simulink library "PC_Simulator_Lib"  (Simulink 8.2)
settings: Solver=ode45  StartTime=0.0  StopTime=10.0  RelTol=1e-3
values from neighbouring files (symbols this model uses):
  data = [r1 r2 r3 r4 L1 L2 L3 L4]    [strasse_Bedatung_HNI_ITI.m]
  distSameLane = 60    [InitialisationsEnv.m]
  eng_speed = [0 60 120 180 240 300 360 420 480 540 600 660 ... (101 elements, 1x101)]    [engine_table.mat]    (also in motor_parameter_calc.m = omega)
  Heading_init = 0    [Start.m]
  inertiaLateral = 25*(radiusWheel)^2    (= 4.129024)    [Start.m]
  laneWidth = 3.6    [InitialisationsEnv.m]    (also in strasse_Bedatung_HNI_ITI.m)
  omega_engine = [0.000000 150.000000 500.000000 1000.000000 1500.000000 2000.000000 2500.000000 3000.000000 3500.000000 4000.000000 4500.000000 5000.000000 5500.000000 6000.000000]    [friction_tables.m]
  omega_max = 6000    [engine_table.mat]    (also in motor_parameter_calc.m)
  omega_wheel = [0 20 40 60 80 100 122 143.7 164]    [friction_tables.m]
  para_Fellow_8_Points = ADAS.Fellow_8_Points    [ADAS_parameters.m]
  position_start_x = [x1 x2 x3 x4 x5 x6 x7]    [strasse_Bedatung_HNI_ITI.m]
  position_start_y = [y1 y2 y3 y4 y5 y6 y7]    [strasse_Bedatung_HNI_ITI.m]
  rad3rdLine = 57.2    [InitialisationsEnv.m]    (also in strasse_Bedatung_HNI_ITI.m)
  radiusWheel = 16*2.54/100    (= 0.4064)    [Start.m]
  s_values = [S1 S2 S3 S4 S5 S6 S7]    [strasse_Bedatung_HNI_ITI.m]
  segmentLimits = [segment1EndThirdLine                   segment2EndThirdLine                   segment3EndThirdLine                   segment4EndThirdLine                   segment5EndThirdLine                   segment6EndThirdLine                   segment7EndThirdLine                   segment8EndThirdLine                   ]    [InitialisationsEnv.m]    (also in strasse_Bedatung_HNI_ITI.m)
  setPosT = [-1.8 -5.4 -1.8 -5.4 -1.8 -5.4 -1.8 -5.4 -1.8 -5.4]    [InitialisationsEnv.m]
  torque = [297.089227105 300.997600937 304.800343044 308.497453426 312.088932082 315.574779014 318.95499422 322.229577701 325.398529457 328.461849487 331.419537793 334.271594373 ... (101 elements, 1x101)]    [engine_table.mat]    (also in motor_parameter_calc.m = g)
  Torque_lost = [0.000000 -8.777780 -15.000000 -26.800000 -29.600000 -32.700000 -35.900000 -39.300000 -42.800000 -46.500000 -50.300000 -54.300000 -58.500000 -62.800000 ]*0.6    [friction_tables.m]
  Torque_lost_wheel = [0.8 0.8 0.75 0.7 0.4 0.3 0.2 0.07 0.07]*0.2    [friction_tables.m]
  X_init = 0    [Start.m]
  Y_init = 1.8    [Start.m]
  Z_init = 0    [Start.m]
undefined symbols (not defined in the file or in its folder): Acc_Pedal, ADAS, Brake_Pedal, Joystick, Newton, Para, Raphson, Standard_Devices, Steering_Wheel_Angle, UDP_Protocol
libraries: simulink x43, rtwinlib x7, dspnetwork x2, simulink_extras x1, vrlib x1
(part 5 of 13)

== system PC_Simulator_Lib/ADAS/Decision_Making_ADAS/Maping_Input ==
  Feedback_ADAS : Inport
  Feedback_Simulationsumgebung : Inport  Port=2
  Abs : Abs
  Bus Selector : BusSelector  OutputSignals=Vehicle_Dynamics.position_CoG.x_CoG[m],Vehicle_Dynamics.position_CoG.y_CoG[m],Vehicle_Dynamics.Oriantation_CoG.Yaw_Angle,Vehicle_Dynamics.Vx_COG[m|s],Environment.Main_Vehicle.t_VUT[m]
  Bus Selector1 : BusSelector  OutputSignals=Unser_Interface_ADAS.ACC.ACC_State,Unser_Interface_ADAS.Pilotiertes_Fahren.Pilotiertes_Fahren_State,Unser_Interface_ADAS.Emergency_Brake.Emergency_Brake_State,Unser_Interface_ADAS.Emergency_Steering.Emergency_Steering_State,Unser_Interface_ADAS.ACC.ACC_Set_Speed[m|s],Unser_Interface_ADAS.ACC.ACC_Time_Gap[s],Sensors_ADAS.Sensors_Front_Out.Object_Detected_In_Lane[bool],Sensors_ADAS.Sensors_Front_Out.Distance[m],Sensors_ADAS.Sensors_Front_Out.Relative_Velocity[m|s],Sensors_ADAS.Sensors_Front_Out.direction_delta_T_available,Sensors_ADAS.Sensors_Front_Out.Lateral_distance_available[m],Sensors_ADAS.Sensors_Front_Out.Heading_Angle_Difference[deg]
  Memory : Memory
  signals_manipulation : Subsystem
  x_CoG_VUT[m] : Outport
  y_CoG_VUT[m] : Outport  Port=2
  yaw_VUT[rad] : Outport  Port=3
  Vx_CoG_VUT[m|s] : Outport  Port=4
  Active_System : Outport  Port=5
  V_User_Set_Speed[m|s] : Outport  Port=6
  Time_Gap[s] : Outport  Port=7
  Object_Inlane[bool] : Outport  Port=8
  Distance_2_Object_Sensor[m] : Outport  Port=9
  v_relative_Sensor[m|s] : Outport  Port=10
  T_current[m] : Outport  Port=11
  Direction_delta_T_Available : Outport  Port=12
  Lateral_Distance_Available[m] : Outport  Port=13
  Heading_Angle_Difference_Absolute[deg] : Outport  Port=14
  wires:
  Abs/1 -> Heading_Angle_Difference_Absolute[deg]/1
  Bus Selector1/12 -> Abs/1  "<Heading_Angle_Difference[deg]>"
  Feedback_Simulationsumgebung/1 -> Bus Selector/1
  Bus Selector/3 -> yaw_VUT[rad]/1  "<Yaw_Angle>"
  Bus Selector/4 -> Vx_CoG_VUT[m|s]/1  "<Vx_COG[m|s]>"
  Bus Selector/2 -> y_CoG_VUT[m]/1  "<y_CoG[m]>"
  Bus Selector/1 -> x_CoG_VUT[m]/1  "<x_CoG[m]>"
  Feedback_ADAS/1 -> Bus Selector1/1
  Bus Selector1/6 -> Time_Gap[s]/1  "<ACC_Time_Gap[s]>"
  Bus Selector1/5 -> Memory/1  "<ACC_Set_Speed[m|s]>"
  Memory/1 -> V_User_Set_Speed[m|s]/1
  Bus Selector1/1 -> signals_manipulation/1(ACC_State)  "<ACC_State>"
  Bus Selector1/7 -> Object_Inlane[bool]/1  "<Object_Detected_In_Lane[bool]>"
  Bus Selector1/8 -> Distance_2_Object_Sensor[m]/1  "<Distance[m]>"
  Bus Selector1/9 -> v_relative_Sensor[m|s]/1  "<Relative_Velocity[m|s]>"
  Bus Selector/5 -> T_current[m]/1  "<t_VUT[m]>"
  Bus Selector1/2 -> signals_manipulation/2(Pilotiertes_Fahren_State)  "<Pilotiertes_Fahren_State>"
  signals_manipulation/1(Active_System) -> Active_System/1
  Bus Selector1/3 -> signals_manipulation/3(Emergency_Brkae_State)  "<Emergency_Brake_State>"
  Bus Selector1/10 -> Direction_delta_T_Available/1  "<direction_delta_T_available>"
  Bus Selector1/11 -> Lateral_Distance_Available[m]/1  "<Lateral_distance_available[m]>"
  Bus Selector1/4 -> signals_manipulation/4(Emergency_Steering_State)  "<Emergency_Steering_State>"

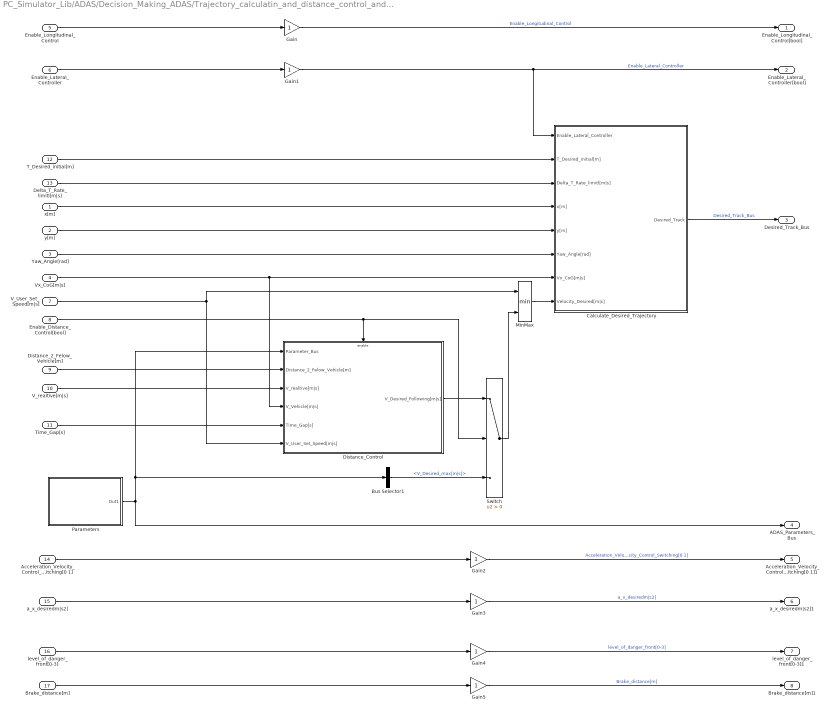
== system PC_Simulator_Lib/ADAS/Decision_Making_ADAS/Trajectory_calculatin_and_distance_control_and output_maping ==
  x[m] : Inport
  y[m] : Inport  Port=2
  Yaw_Angle[rad] : Inport  Port=3
  Vx_CoG[m|s] : Inport  Port=4
  Enable_Longitudinal_Control : Inport  Port=5
  Enable_Lateral_Controller : Inport  Port=6
  V_User_Set_Speed[m|s] : Inport  Port=7
  Enable_Distance_Control[bool] : Inport  Port=8
  Distance_2_Felow_Vehicle[m] : Inport  Port=9
  V_realtive[m|s] : Inport  Port=10
  Time_Gap[s] : Inport  Port=11
  T_Desired_initial[m] : Inport  Port=12
  Delta_T_Rate_limitl[m|s] : Inport  Port=13
  Acceleration_Velocity_Control_Switching[0 1] : Inport  Port=14
  a_x_desiredm|s2] : Inport  Port=15
  level_of_danger_front[0-3] : Inport  Port=16
  Brake_distance[m] : Inport  Port=17
  Bus Selector1 : BusSelector  OutputSignals=V_Desired_max[m|s]
  Calculate_Desired_Trajectory : Subsystem
  Distance_Control : Subsystem
  Gain{,1..5} (6 alike) : Gain
  MinMax : MinMax  Inputs=2
  Parameters : Subsystem
  Switch : Switch  Criteria=u2 > Threshold
  Enable_Longitudinal_Control[bool] : Outport
  Enable_Lateral_Controller[bool] : Outport  Port=2
  Desired_Track_Bus : Outport  Port=3
  ADAS_Parameters_Bus : Outport  Port=4
  Acceleration_Velocity_Control_Switching[0 1]1 : Outport  Port=5
  "a_x_desiredm|s2]1 " : Outport  Port=6
  level_of_danger_front[0-3]1 : Outport  Port=7
  Brake_distance[m]1 : Outport  Port=8
  wires:
  Brake_distance[m]/1 -> Gain5/1
  Gain5/1 -> Brake_distance[m]1/1  "Brake_distance[m]"
  Gain4/1 -> level_of_danger_front[0-3]1/1  "level_of_danger_front[0-3]"
  level_of_danger_front[0-3]/1 -> Gain4/1
  Enable_Lateral_Controller/1 -> Gain1/1
  V_realtive[m|s]/1 -> Distance_Control/3(V_realtive[m|s])
  V_User_Set_Speed[m|s]/1 -> MinMax/1, Distance_Control/6(V_User_Set_Speed[m|s])
  T_Desired_initial[m]/1 -> Calculate_Desired_Trajectory/2(T_Desired_initial[m])
  Delta_T_Rate_limitl[m|s]/1 -> Calculate_Desired_Trajectory/3(Delta_T_Rate_limitl[m|s])
  Enable_Longitudinal_Control/1 -> Gain/1
  Calculate_Desired_Trajectory/1(Desired_Track) -> Desired_Track_Bus/1  "Desired_Track_Bus"
  MinMax/1 -> Calculate_Desired_Trajectory/8(Velocity_Desired[m|s])
  Distance_Control/1(V_Desired_Following[m|s]) -> Switch/1
  Enable_Distance_Control[bool]/1 -> Switch/2, Distance_Control/Enable
  Bus Selector1/1 -> Switch/3  "<V_Desired_max[m|s]>"
  Switch/1 -> MinMax/2
  Time_Gap[s]/1 -> Distance_Control/5(Time_Gap[s])
  x[m]/1 -> Calculate_Desired_Trajectory/4(x[m])
  y[m]/1 -> Calculate_Desired_Trajectory/5(y[m])
  Vx_CoG[m|s]/1 -> Calculate_Desired_Trajectory/7(Vx_CoG[m|s]), Distance_Control/4(V_Vehicle[m|s])
  Yaw_Angle[rad]/1 -> Calculate_Desired_Trajectory/6(Yaw_Angle[rad])
  Parameters/1(Out1) -> ADAS_Parameters_Bus/1, Distance_Control/1(Parameter_Bus), Bus Selector1/1
  Distance_2_Felow_Vehicle[m]/1 -> Distance_Control/2(Distance_2_Felow_Vehicle[m])
  Gain/1 -> Enable_Longitudinal_Control[bool]/1  "Enable_Longitudinal_Control"
  Gain1/1 -> Enable_Lateral_Controller[bool]/1, Calculate_Desired_Trajectory/1(Enable_Lateral_Controller)  "Enable_Lateral_Controller"
  Acceleration_Velocity_Control_Switching[0 1]/1 -> Gain2/1
  Gain2/1 -> Acceleration_Velocity_Control_Switching[0 1]1/1  "Acceleration_Velocity_Control_Switching[0 1]"
  a_x_desiredm|s2]/1 -> Gain3/1
  Gain3/1 -> "a_x_desiredm|s2]1 "/1  "a_x_desiredm|s2]"

== system PC_Simulator_Lib/ADAS/Execution_ADAS/Input_Interface ==
  Feedback_ADAS : Inport
  Feedback_Simulationsumgebung : Inport  Port=2
  Bus Selector : BusSelector  OutputSignals=Vehicle_Dynamics.ax_COG[m|s2],Vehicle_Dynamics.Vx_COG[m|s],Drive_Train.Omega_4_Wheels[rad|s],Drive_Train.Omega_Engine[rad|s],Drive_Train.Gearbox_Gear_Ratio,Driver_Interface.Acc_Pedal_norm,Driver_Interface.Brake_Pedal_norm,Driver_Interface.Steering_wheel_norm,Vehicle_Dynamics.Vy_COG[m|s],Vehicle_Dynamics.Oriantation_CoG.Yaw_Angle,Vehicle_Dynamics.Yaw_Rate[rad|s],Vehicle_Dynamics.position_CoG.x_CoG[m],Vehicle_Dynamics.position_CoG.y_CoG[m]
  Bus Selector1 : BusSelector  OutputSignals=Decision_Making_ADAS.Enable_Longitudinal_Control,Decision_Making_ADAS.Enable_Lateral_Controller,Decision_Making_ADAS.Desired_Track_Bus.x_Desired[m],Decision_Making_ADAS.Desired_Track_Bus.y_Desired[m],Decision_Making_ADAS.Desired_Track_Bus.Velocity_Desired[m|s],Decision_Making_ADAS.Desired_Track_Bus.acceleration_Desired[m|s2],Decision_Making_ADAS.Desired_Track_Bus.Heading_angle_Desired[rad],Decision_Making_ADAS.Desired_Track_Bus.Curvature_Desired_Track[1|m],Decision_Making_ADAS.ADAS_Parameters.acceleration_max[m|s2],Decision_Making_ADAS.ADAS_Parameters.acceleration_min[m|s2],Decision_Making_ADAS.Acceleration_Velocity_Control_Switching[0 1],Decision_Making_ADAS.a_x_desiredm|s2]
  Differential_Gear_Ratio1 : Constant  Value=Para.DT.Differential_Gear_ratio.v
  a_x_actual[m|s2] : Outport
  Vx_CoG[m|s] : Outport  Port=2
  Omega_4_Wheels[rad|s] : Outport  Port=3
  Omega_Engine[rad|s] : Outport  Port=4
  Gearbox_Gear_Ratio : Outport  Port=5
  Differential_Gear_Ratio : Outport  Port=6
  acceleration_max[m|s2] : Outport  Port=7
  acceleration_min[m|s2] : Outport  Port=8
  Acceleration_Velocity_Control_Switching[0 1] : Outport  Port=9
  a_x_desired[m|s2] : Outport  Port=10
  Eanbel_Longitudidinal_Controller : Outport  Port=11
  Eanbel_Lateral_Controller : Outport  Port=12
  Acc_Pedal_user[norm] : Outport  Port=13
  Brake_Pedal_user[norm] : Outport  Port=14
  Steering_Wheel_Angle[norm] : Outport  Port=15
  Vy_CoG[m|s] : Outport  Port=16
  Yaw_Angle[rad] : Outport  Port=17
  Yaw_Rate[rad|s] : Outport  Port=18
  x_CoG[m] : Outport  Port=19
  y_CoG[m] : Outport  Port=20
  x_Desired[m] : Outport  Port=21
  y_Desired[m] : Outport  Port=22
  Velocity_Desired[m|s] : Outport  Port=23
  acceleration_Desired[m|s2] : Outport  Port=24
  Heading_Angle_Desired[rad] : Outport  Port=25
  Curvature_Desired_Track[1|m] : Outport  Port=26
  wires:
  Feedback_Simulationsumgebung/1 -> Bus Selector/1
  Bus Selector/1 -> a_x_actual[m|s2]/1  "<ax_COG[m|s2]>"
  Bus Selector/2 -> Vx_CoG[m|s]/1  "<Vx_COG[m|s]>"
  Differential_Gear_Ratio1/1 -> Differential_Gear_Ratio/1
  Bus Selector/3 -> Omega_4_Wheels[rad|s]/1  "<Omega_4_Wheels[rad|s]>"
  Bus Selector/4 -> Omega_Engine[rad|s]/1  "<Omega_Engine[rad|s]>"
  Bus Selector/5 -> Gearbox_Gear_Ratio/1  "<Gearbox_Gear_Ratio>"
  Feedback_ADAS/1 -> Bus Selector1/1
  Bus Selector1/1 -> Eanbel_Longitudidinal_Controller/1  "<Enable_Longitudinal_Control>"
  Bus Selector/6 -> Acc_Pedal_user[norm]/1  "<Acc_Pedal_norm>"
  Bus Selector/7 -> Brake_Pedal_user[norm]/1  "<Brake_Pedal_norm>"
  Bus Selector/8 -> Steering_Wheel_Angle[norm]/1  "<Steering_wheel_norm>"
  Bus Selector/9 -> Vy_CoG[m|s]/1  "<Vy_COG[m|s]>"
  Bus Selector/10 -> Yaw_Angle[rad]/1  "<Yaw_Angle>"
  Bus Selector/11 -> Yaw_Rate[rad|s]/1  "<Yaw_Rate[rad|s]>"
  Bus Selector/12 -> x_CoG[m]/1  "<x_CoG[m]>"
  Bus Selector/13 -> y_CoG[m]/1  "<y_CoG[m]>"
  Bus Selector1/3 -> x_Desired[m]/1  "<x_Desired[m]>"
  Bus Selector1/5 -> Velocity_Desired[m|s]/1  "<Velocity_Desired[m|s]>"
  Bus Selector1/4 -> y_Desired[m]/1  "<y_Desired[m]>"
  Bus Selector1/6 -> acceleration_Desired[m|s2]/1  "<acceleration_Desired[m|s2]>"
  Bus Selector1/7 -> Heading_Angle_Desired[rad]/1  "<Heading_angle_Desired[rad]>"
  Bus Selector1/8 -> Curvature_Desired_Track[1|m]/1  "<Curvature_Desired_Track[1|m]>"
  Bus Selector1/10 -> acceleration_min[m|s2]/1  "<acceleration_min[m|s2]>"
  Bus Selector1/9 -> acceleration_max[m|s2]/1  "<acceleration_max[m|s2]>"
  Bus Selector1/2 -> Eanbel_Lateral_Controller/1  "<Enable_Lateral_Controller>"
  Bus Selector1/11 -> Acceleration_Velocity_Control_Switching[0 1]/1  "<Acceleration_Velocity_Control_Switching[0 1]>"
  Bus Selector1/12 -> a_x_desired[m|s2]/1  "<a_x_desiredm|s2]>"

== system PC_Simulator_Lib/ADAS/Execution_ADAS/Lateral_Controller_S_Function ==
  Vx_CoG[m|s] : Inport
  Vy_CoG[m|s] : Inport  Port=2
  Yaw_Angle[rad] : Inport  Port=3
  Yaw_Rate[rad|s] : Inport  Port=4
  x_CoG[m] : Inport  Port=5
  y_CoG[m] : Inport  Port=6
  x_Desired[m] : Inport  Port=7
  y_Desired[m] : Inport  Port=8
  Velocity_Desired[m|s] : Inport  Port=9
  acceleration_Desired[m|s2] : Inport  Port=10
  Heading_Angle_Desired[rad] : Inport  Port=11
  Curvature_Desired_Track[1|m] : Inport  Port=12
  Enable : EnablePort  StatesWhenEnabling=reset
  Lateral_controller : Subsystem
  Product : Product
  calculate_slip_ange_and_absolute_velocity : Subsystem
  Steering_Wheel_Angle[norm] : Outport
  wires:
  Yaw_Rate[rad|s]/1 -> Lateral_controller/6(Yaw_Rate)
  x_CoG[m]/1 -> Lateral_controller/1(x_CoG_Global)
  Velocity_Desired[m|s]/1 -> Lateral_controller/11(v_Desired)
  acceleration_Desired[m|s2]/1 -> Lateral_controller/12(a_Desired)
  Heading_Angle_Desired[rad]/1 -> Lateral_controller/9(Yaw_Desired)
  Curvature_Desired_Track[1|m]/1 -> Product/2
  y_Desired[m]/1 -> Lateral_controller/8(y_Desired)
  x_Desired[m]/1 -> Lateral_controller/7(x_Desire)
  calculate_slip_ange_and_absolute_velocity/2(Slip_Angle[rad]) -> Lateral_controller/4(Slip_Angle)
  Vx_CoG[m|s]/1 -> calculate_slip_ange_and_absolute_velocity/1(Vx_CoG[m|s])
  Vy_CoG[m|s]/1 -> calculate_slip_ange_and_absolute_velocity/2(Vy_CoG[m|s])
  Product/1 -> Lateral_controller/10(Yaw_Rate_Desired)
  calculate_slip_ange_and_absolute_velocity/1(v_CoG[m|s]) -> Product/1, Lateral_controller/3(v_CoG)
  y_CoG[m]/1 -> Lateral_controller/2(y_CoG_Global)
  Lateral_controller/1(Steering_Wheel_Angle[norm]) -> Steering_Wheel_Angle[norm]/1
  Yaw_Angle[rad]/1 -> Lateral_controller/5(Yaw_Angle)

== system PC_Simulator_Lib/ADAS/Execution_ADAS/Longitudinal_Controller ==
  Vx_desired[m|s] : Inport
  a_acctual[m|s2] : Inport  Port=2
  Vx_CoG[m|s] : Inport  Port=3
  omega_4_Wheels[rad|s] : Inport  Port=4
  Omega_Engine[rad|s] : Inport  Port=5
  Gearbox_Gear_Ratio : Inport  Port=6
  Differential_Gear_Ratio : Inport  Port=7
  acceleration_max[m|s2] : Inport  Port=8
  acceleration_min[m|s2] : Inport  Port=9
  Acceleration_Velocity_Control_Switching[0|1] : Inport  Port=10
  ax_desired[m|s2] : Inport  Port=11
  Enable : EnablePort
  Acceleration_Control : Subsystem
  Switch : Switch  Criteria=u2 > Threshold
  Velocity_Control : Subsystem
  Acc_Pedal[norm] : Outport
  Brake_Pedal[norm] : Outport  Port=2
  wires:
  Acceleration_Control/1(Gas_Pedal[norm]) -> Acc_Pedal[norm]/1
  a_acctual[m|s2]/1 -> Acceleration_Control/2(a_acctual[m|s2])
  omega_4_Wheels[rad|s]/1 -> Acceleration_Control/4(omega_4_Wheels[rad|s])
  Gearbox_Gear_Ratio/1 -> Acceleration_Control/6(Gearbox_Gear_Ratio)
  Differential_Gear_Ratio/1 -> Acceleration_Control/7(Differential_Gear_Ratio)
  Omega_Engine[rad|s]/1 -> Acceleration_Control/5(Omega_Engine[rad|s])
  Vx_CoG[m|s]/1 -> Velocity_Control/2(Vx_acctual[m|s]), Acceleration_Control/3(Vx_CoG[m|s])
  Acceleration_Control/2(Brake_Pedal[norm]) -> Brake_Pedal[norm]/1
  Vx_desired[m|s]/1 -> Velocity_Control/1(Vx_desired[m|s])
  acceleration_min[m|s2]/1 -> Velocity_Control/4(acceleration_min[m|s2])
  acceleration_max[m|s2]/1 -> Velocity_Control/3(acceleration_max[m|s2])
  Acceleration_Velocity_Control_Switching[0|1]/1 -> Velocity_Control/Enable, Switch/2
  Switch/1 -> Acceleration_Control/1(a_desired[m|s2])
  ax_desired[m|s2]/1 -> Switch/3
  Velocity_Control/1(a_desired[m|s2]) -> Switch/1

== system PC_Simulator_Lib/ADAS/Execution_ADAS/Output_Interface ==
  Acc_Pedal[norm] : Inport
  Brake_Pedal[norm] : Inport  Port=2
  Eanbel_Longitudidinal_Controller : Inport  Port=3
  Eanbel_Lateral_Controller : Inport  Port=4
  Acc_Pedal_user[norm] : Inport  Port=5
  Brake_Pedal_user[norm] : Inport  Port=6
  Steering_Wheel_Angle_Controller[norm] : Inport  Port=7
  Steering_Wheel_Angle_User[norm] : Inport  Port=8
  Bus Assignment : BusAssignment  AssignedSignals=Acc_Pedal[norm],Brake_Pedal[norm],Steering_Wheel_Angle[norm]
  Bus Creator : BusCreator  Inputs=3
  Bus Creator1 : BusCreator  Inputs=2
  Gain : Gain
  Gain1 : Gain
  Gain2 : Gain
  Subsystem : Subsystem
  Out1 : Outport
  wires:
  Bus Creator1/1 -> Out1/1
  Acc_Pedal[norm]/1 -> Gain/1
  Bus Creator/1 -> Bus Assignment/1, Bus Creator1/2  "ADAS_controller_values"
  Bus Assignment/1 -> Bus Creator1/1  "actions_on_vehicle"
  Brake_Pedal[norm]/1 -> Gain1/1
  Gain/1 -> Subsystem/1(Acc_Pedal_ADAS[norm]), Bus Creator/1  "Acc_Pedal[norm]"
  Gain1/1 -> Subsystem/2(Brake_Pedal__ADAS[norm]), Bus Creator/2  "Brake_Pedal[norm]"
  Steering_Wheel_Angle_Controller[norm]/1 -> Gain2/1
  Gain2/1 -> Subsystem/3(Steering_Wheel_Angle_ADAS[norm]), Bus Creator/3  "Steering_Wheel_Angle[norm]"
  Subsystem/1(Acc_Pedal[norm]) -> Bus Assignment/2
  Subsystem/2(Brake_Pedal[norm]) -> Bus Assignment/3
  Subsystem/3(Steering_Wheel_Angle[norm]) -> Bus Assignment/4
  Brake_Pedal_user[norm]/1 -> Subsystem/7(Brake_Pedal_user[norm])
  Acc_Pedal_user[norm]/1 -> Subsystem/6(Acc_Pedal_user[norm])
  Steering_Wheel_Angle_User[norm]/1 -> Subsystem/8(Steering_Wheel_Angle_User[norm])
  Eanbel_Longitudidinal_Controller/1 -> Subsystem/4(Eanbel_Longitudidinal_Controller)
  Eanbel_Lateral_Controller/1 -> Subsystem/5(Eanbel_Lateral_Controller)

== system PC_Simulator_Lib/ADAS/Sensors_ADAS/Front_Long_Range_Radar_Sensor ==
  Position_VUT_Vector[m] : Inport
  Oriantation_VUT_Vector[rad] : Inport  Port=2
  Position_Fellows[m] : Inport  Port=3
  Oriantation_Fellows[rad] : Inport  Port=4
  Constant1 : Constant  Value=ADAS.Front_Long_Range_Radar.Fellow_size
  Coordinate_TRansformation_of_Fellows_Points_Plus_Calculation_Distances_And_Angles : Subsystem
  First_STage_Coordinate_Transformation : Subsystem
  Intersection_Detection : Subsystem
  Objects_Dectected_LRR[bool] : Outport
  delta_s_Vector_LRR[m] : Outport  Port=2
  Angle_Horizontal_Vector_LRR[rad] : Outport  Port=3
  Positon_of_detected_Points_LRR[m] : Outport  Port=4
  wires:
  First_STage_Coordinate_Transformation/5(Round_done[bool]) -> Intersection_Detection/6(Round_done[bool])
  Position_VUT_Vector[m]/1 -> First_STage_Coordinate_Transformation/1(Position_VUT_Vector[m])
  Oriantation_VUT_Vector[rad]/1 -> First_STage_Coordinate_Transformation/2(Oriantation_VUT_Vector[rad]), Coordinate_TRansformation_of_Fellows_Points_Plus_Calculation_Distances_And_Angles/3(Oriantation_VUT_Vector[rad])
  First_STage_Coordinate_Transformation/1(Upper_Triangles_Vector[m]) -> Intersection_Detection/2(Tiangle_upper_Points_Vetctor[m])
  First_STage_Coordinate_Transformation/2(Centeral_Triangles_Vector[m]) -> Intersection_Detection/3(Tiangle_Center_Points_Vetctor[m])
  First_STage_Coordinate_Transformation/3(Lower_Triangles_Vector[m]) -> Intersection_Detection/4(Tiangle_Lower_Points_Vetctor[m])
  First_STage_Coordinate_Transformation/4(Inside_Sphere_Vector[bool]) -> Intersection_Detection/5(Inside_Sphere_Vector[bool])
  Intersection_Detection/1(Objects_Dectected[bool]) -> Coordinate_TRansformation_of_Fellows_Points_Plus_Calculation_Distances_And_Angles/1(Objects_Dectected[bool]), Objects_Dectected_LRR[bool]/1  "Objects_Dectected[bool]"
  Constant1/1 -> Intersection_Detection/1(Cuboid_Dimentions_vector[m])
  First_STage_Coordinate_Transformation/6(Apex_Position_Global[m]) -> Coordinate_TRansformation_of_Fellows_Points_Plus_Calculation_Distances_And_Angles/2(Apex_Pos_Global[m])
  Coordinate_TRansformation_of_Fellows_Points_Plus_Calculation_Distances_And_Angles/2(Angle_Horizontal_Vector[rad]) -> Angle_Horizontal_Vector_LRR[rad]/1  "Angle_Horizontal_Vector[rad]"
  Coordinate_TRansformation_of_Fellows_Points_Plus_Calculation_Distances_And_Angles/1(delta_s_Vector[m]) -> delta_s_Vector_LRR[m]/1  "delta_s_Vector[m]"
  Coordinate_TRansformation_of_Fellows_Points_Plus_Calculation_Distances_And_Angles/3(Positon_of_detected_Points[m]) -> Positon_of_detected_Points_LRR[m]/1
  Position_Fellows[m]/1 -> First_STage_Coordinate_Transformation/3(Position_Fellows[m]), Coordinate_TRansformation_of_Fellows_Points_Plus_Calculation_Distances_And_Angles/4(Position_Fellows[m])
  Oriantation_Fellows[rad]/1 -> First_STage_Coordinate_Transformation/4(Oriantation_Fellows[rad]), Coordinate_TRansformation_of_Fellows_Points_Plus_Calculation_Distances_And_Angles/5(Oriantation_Fellows[rad])

== system PC_Simulator_Lib/ADAS/Sensors_ADAS/Front_Mid_Range_Radar_Sensor ==
  Position_VUT_Vector[m] : Inport
  Oriantation_VUT_Vector[rad] : Inport  Port=2
  Position_Fellows[m] : Inport  Port=3
  Oriantation_Fellows[rad] : Inport  Port=4
  Constant1 : Constant  Value=ADAS.Front_Long_Range_Radar.Fellow_size
  Coordinate_TRansformation_of_Fellows_Points_Plus_Calculation_Distances_And_Angles : Subsystem
  First_STage_Coordinate_Transformation : Subsystem
  Intersection_Detection : Subsystem
  Objects_Dectected_MRR[bool] : Outport
  delta_s_Vector_MRR[m] : Outport  Port=2
  Angle_Horizontal_Vector_MRR[rad] : Outport  Port=3
  Positon_of_detected_Points_MRR[m] : Outport  Port=4
  wires:
  First_STage_Coordinate_Transformation/5(Round_simulation_time[ms]) -> Intersection_Detection/6(Round_simulation_time[ms])
  Position_VUT_Vector[m]/1 -> First_STage_Coordinate_Transformation/1(Position_VUT_Vector[m])
  Oriantation_VUT_Vector[rad]/1 -> Coordinate_TRansformation_of_Fellows_Points_Plus_Calculation_Distances_And_Angles/3(Oriantation_VUT_Vector[rad]), First_STage_Coordinate_Transformation/2(Oriantation_VUT_Vector[rad])
  First_STage_Coordinate_Transformation/1(Upper_Triangles_Vector[m]) -> Intersection_Detection/2(Tiangle_upper_Points_Vetctor[m])
  First_STage_Coordinate_Transformation/2(Centeral_Triangles_Vector[m]) -> Intersection_Detection/3(Tiangle_Center_Points_Vetctor[m])
  First_STage_Coordinate_Transformation/3(Lower_Triangles_Vector[m]) -> Intersection_Detection/4(Tiangle_Lower_Points_Vetctor[m])
  First_STage_Coordinate_Transformation/4(Inside_Sphere_Vector[bool]) -> Intersection_Detection/5(Inside_Sphere_Vector[bool])
  Intersection_Detection/1(Objects_Dectected[bool]) -> Coordinate_TRansformation_of_Fellows_Points_Plus_Calculation_Distances_And_Angles/1(Objects_Dectected[bool]), Objects_Dectected_MRR[bool]/1  "Objects_Dectected[bool]"
  Constant1/1 -> Intersection_Detection/1(Cuboid_Dimentions_vector[m])
  First_STage_Coordinate_Transformation/6(Apex_Position_Global[m]) -> Coordinate_TRansformation_of_Fellows_Points_Plus_Calculation_Distances_And_Angles/2(Apex_Pos_Global[m])
  Coordinate_TRansformation_of_Fellows_Points_Plus_Calculation_Distances_And_Angles/2(Angle_Horizontal_Vector[rad]) -> Angle_Horizontal_Vector_MRR[rad]/1  "Angle_Horizontal_Vector[rad]"
  Coordinate_TRansformation_of_Fellows_Points_Plus_Calculation_Distances_And_Angles/1(delta_s_Vector[m]) -> delta_s_Vector_MRR[m]/1  "delta_s_Vector[m]"
  Coordinate_TRansformation_of_Fellows_Points_Plus_Calculation_Distances_And_Angles/3(Positon_of_detected_Points[m]) -> Positon_of_detected_Points_MRR[m]/1
  Position_Fellows[m]/1 -> Coordinate_TRansformation_of_Fellows_Points_Plus_Calculation_Distances_And_Angles/4(Position_Fellows[m]), First_STage_Coordinate_Transformation/3(Position_Fellows[m])
  Oriantation_Fellows[rad]/1 -> Coordinate_TRansformation_of_Fellows_Points_Plus_Calculation_Distances_And_Angles/5(Oriantation_Fellows[rad]), First_STage_Coordinate_Transformation/4(Oriantation_Fellows[rad])

== system PC_Simulator_Lib/ADAS/Sensors_ADAS/Input_Maping ==
  Feedback_ADAS : Inport
  Feedback_Simulationsumgebung : Inport  Port=2
  Fellows : Subsystem
  Terminator : Terminator
  VUT : Subsystem
  Position_Global_VUT_Vector[m] : Outport
  Oriantation_VUT_Vector[rad] : Outport  Port=2
  Position_Fellows[m] : Outport  Port=3
  Oriantation_Fellows[rad] : Outport  Port=4
  wires:
  VUT/2(Oriantation_VUT_Vector[rad]) -> Oriantation_VUT_Vector[rad]/1
  Feedback_ADAS/1 -> Terminator/1
  Feedback_Simulationsumgebung/1 -> Fellows/1(Feedback_Simulationsumgebung), VUT/1(Feedback_Simulationsumgebung)
  Fellows/1(Position_Fellows[m]) -> Position_Fellows[m]/1
  Fellows/2(Oriantation_Fellows[rad]) -> Oriantation_Fellows[rad]/1
  VUT/1(Position_Global_VUT_Vector[m]) -> Position_Global_VUT_Vector[m]/1

== system PC_Simulator_Lib/ADAS/Sensors_ADAS/Object_Selection_Based_On_LRR_MRR_and_Camera SENSOR FUSION ==
  Objects_Dectected_LRR[bool] : Inport
  delta_s_Vector_LRR[m] : Inport  Port=2
  Angle_Horizontal_Vector_LRR[rad] : Inport  Port=3
  T_Detected_Points_LRR[m] : Inport  Port=4
  Objects_Dectected_MRR[bool] : Inport  Port=5
  delta_s_Vector_MRR[m] : Inport  Port=6
  Angle_Horizontal_Vector_MRR[rad] : Inport  Port=7
  T_Detected_Points_MRR[m] : Inport  Port=8
  T_VUT[m] : Inport  Port=9
  Heading_Angle_Road_under_VUT[deg] : Inport  Port=10
  Yaw_Angle_VUT[rad] : Inport  Port=11
  Bus Creator : BusCreator  Inputs=6
  Constant : Constant  Value=360
  Derivative : Derivative
  Gain1 : Gain  Gain=180/pi
  MATLAB Function : MATLAB Function  TreatAsAtomicUnit=on
  Math Function : Math  Operator=rem  SaturateOnIntegerOverflow=on
  Rate Limiter : RateLimiter  RisingSlewLimit=200  FallingSlewLimit=-200  SampleTimeMode=inherited
  Subtract : Sum  Inputs=+-
  Sensors_Front_Out : Outport
  wires:
  Constant/1 -> Math Function/2
  Math Function/1 -> Subtract/2
  Subtract/1 -> Bus Creator/6  "Heading_Angle_Difference[deg]"
  Heading_Angle_Road_under_VUT[deg]/1 -> Subtract/1
  Yaw_Angle_VUT[rad]/1 -> Gain1/1
  Gain1/1 -> Math Function/1
  Bus Creator/1 -> Sensors_Front_Out/1
  Objects_Dectected_LRR[bool]/1 -> MATLAB Function/1(objects_dectected_LRR)
  delta_s_Vector_LRR[m]/1 -> MATLAB Function/2(delta_s_vector_LRR)
  MATLAB Function/1(object_in_lane) -> Bus Creator/1  "Object_Detected_In_Lane[bool]"
  T_Detected_Points_LRR[m]/1 -> MATLAB Function/4(T_Objects_LRR)
  Angle_Horizontal_Vector_LRR[rad]/1 -> MATLAB Function/3(angle_H_vector_LRR)
  T_VUT[m]/1 -> MATLAB Function/9(T_VUT)
  Derivative/1 -> Rate Limiter/1
  Rate Limiter/1 -> Bus Creator/3  "Relative_Velocity[m|s]"
  MATLAB Function/2(distance) -> Derivative/1, Bus Creator/2  "Distance[m]"
  Objects_Dectected_MRR[bool]/1 -> MATLAB Function/5(objects_dectected_MRR)
  delta_s_Vector_MRR[m]/1 -> MATLAB Function/6(delta_s_vector_MRR)
  Angle_Horizontal_Vector_MRR[rad]/1 -> MATLAB Function/7(angle_H_vector_MRR)
  T_Detected_Points_MRR[m]/1 -> MATLAB Function/8(T_Objects_MRR)
  MATLAB Function/3(direction_delta_T) -> Bus Creator/4  "direction_delta_T_available"
  MATLAB Function/4(distance_lateral) -> Bus Creator/5  "Lateral_distance_available[m]"

== system PC_Simulator_Lib/ADAS/Sensors_ADAS/Output_Mapint ==
  Sensors_Front_Out : Inport
  Bus Creator : BusCreator  Inputs=1
  Sensors_Output : Outport
  wires:
  Bus Creator/1 -> Sensors_Output/1
  Sensors_Front_Out/1 -> Bus Creator/1  "Sensors_Front_Out"

== system PC_Simulator_Lib/ADAS/Sensors_ADAS/convert_xy_2_st ==
  Positon_of_detected_Points_LRR[m] : Inport
  Constant : Constant  Value=data
  Constant1 : Constant  Value=position_start_x
  Constant2 : Constant  Value=position_start_y
  Constant3 : Constant  Value=s_values
  Embedded MATLAB Function : MATLAB Function  TreatAsAtomicUnit=on
  Terminator{1..4} (4 alike) : Terminator
  T_Detected_Points_LRR[m] : Outport
  wires:
  Constant/1 -> Embedded MATLAB Function/1(data)
  Constant1/1 -> Embedded MATLAB Function/2(position_start_x)
  Constant2/1 -> Embedded MATLAB Function/3(position_start_y)
  Constant3/1 -> Embedded MATLAB Function/4(s_values)
  Embedded MATLAB Function/3(mue) -> Terminator2/1
  Embedded MATLAB Function/1(z) -> Terminator3/1
  Positon_of_detected_Points_LRR[m]/1 -> Embedded MATLAB Function/5(Positon_of_detected_Points)
  Embedded MATLAB Function/4(s) -> Terminator4/1
  Embedded MATLAB Function/5(t) -> T_Detected_Points_LRR[m]/1
  Embedded MATLAB Function/2(psi) -> Terminator1/1

== system PC_Simulator_Lib/ADAS/Sensors_ADAS/convert_xy_2_st1 ==
  Positon_of_detected_Points[m] : Inport
  Constant : Constant  Value=data
  Constant1 : Constant  Value=position_start_x
  Constant2 : Constant  Value=position_start_y
  Constant3 : Constant  Value=s_values
  Embedded MATLAB Function : MATLAB Function  TreatAsAtomicUnit=on
  Terminator{1..4} (4 alike) : Terminator
  T_Detected_Points[m] : Outport
  wires:
  Embedded MATLAB Function/2(psi) -> Terminator1/1
  Embedded MATLAB Function/5(t) -> T_Detected_Points[m]/1
  Embedded MATLAB Function/4(s) -> Terminator4/1
  Positon_of_detected_Points[m]/1 -> Embedded MATLAB Function/5(Positon_of_detected_Points)
  Embedded MATLAB Function/1(z) -> Terminator3/1
  Embedded MATLAB Function/3(mue) -> Terminator2/1
  Constant3/1 -> Embedded MATLAB Function/4(s_values)
  Constant2/1 -> Embedded MATLAB Function/3(position_start_y)
  Constant1/1 -> Embedded MATLAB Function/2(position_start_x)
  Constant/1 -> Embedded MATLAB Function/1(data)

== system PC_Simulator_Lib/ADAS/Unser_Interface_ADAS/ACC_User_Interface ==
  Feedback_ADAS : Inport
  Feedback_Simulationsumgebung : Inport  Port=2
  ACC_User_Control : Stateflow chart  TreatAsAtomicUnit=on
  Bus Selector : BusSelector  OutputSignals=Driver_Interface.ACC_Plus_Button,Driver_Interface.ACC_Minus_Button,Driver_Interface.ACC_Stop_Button,Driver_Interface.ACC_Resume_Button
  Bus Selector1 : BusSelector  OutputSignals=Driver_Interface.DNR,Driver_Interface.Acc_Pedal_norm,Driver_Interface.Brake_Pedal_norm,Vehicle_Dynamics.Vx_COG[m|s]
  Bus Selector2 : BusSelector  OutputSignals=Driver_Interface.Time_Gap_Mode_Switching_Button
  Bus Selector3 : BusSelector  OutputSignals=Unser_Interface_ADAS.Pilotiertes_Fahren.Pilotiertes_Fahren_State,Unser_Interface_ADAS.Emergency_Brake.Emergency_Brake_State,Unser_Interface_ADAS.Emergency_Steering.Emergency_Steering_State
  Bus Selector4 : BusSelector  OutputSignals=Execution_ADAS.ADAS_controller_values.Acc_Pedal[norm],Execution_ADAS.ADAS_controller_values.Brake_Pedal[norm]
  Logical Operator : Logic  Operator=OR  Inputs=3  AllPortsSameDT=off  OutDataTypeStr=boolean
  Memory : Memory
  Memory1 : Memory
  Memory2 : Memory
  Mux : Mux  Inputs=5
  Mux1 : Mux  Inputs=2
  Pulse Generator : DiscretePulseGenerator  PulseType=Time based  Period=0.1  PulseWidth=50
  Time_Gap_switching : Stateflow chart  TreatAsAtomicUnit=on
  ACC_State[bool] : Outport
  ACC_Set_Speed[m|s] : Outport  Port=2
  ACC_Time_Gap_Mode[1-3] : Outport  Port=3
  wires:
  Bus Selector4/2 -> ACC_User_Control/6(Brake_Pedal_ACC)  "<Brake_Pedal[norm]>"
  Bus Selector4/1 -> ACC_User_Control/5(Gas_Pedal_ACC)  "<Acc_Pedal[norm]>"
  ACC_User_Control/1(ACC_State) -> ACC_State[bool]/1
  Bus Selector1/1 -> ACC_User_Control/1(Gearbox_State)  "<DNR>"
  Bus Selector1/2 -> ACC_User_Control/2(Gas_Pedal_User)  "<Acc_Pedal_norm>"
  Bus Selector1/3 -> ACC_User_Control/3(Brake_Pedal_User)  "<Brake_Pedal_norm>"
  Mux/1 -> ACC_User_Control/Trigger
  ACC_User_Control/2(Set_Speed) -> ACC_Set_Speed[m|s]/1
  Feedback_Simulationsumgebung/1 -> Bus Selector1/1, Bus Selector2/1, Bus Selector/1
  Bus Selector/4 -> Mux/5  "<ACC_Resume_Button>"
  Bus Selector/3 -> Mux/4  "<ACC_Stop_Button>"
  Bus Selector/2 -> Mux/3  "<ACC_Minus_Button>"
  Bus Selector/1 -> Mux/2  "<ACC_Plus_Button>"
  Bus Selector1/4 -> ACC_User_Control/4(Velocity_VUT)  "<Vx_COG[m|s]>"
  Time_Gap_switching/1(Time_Gap) -> ACC_Time_Gap_Mode[1-3]/1
  Mux1/1 -> Time_Gap_switching/Trigger
  Pulse Generator/1 -> Mux1/1, Mux/1
  Bus Selector2/1 -> Mux1/2  "<Time_Gap_Mode_Switching_Button>"
  Bus Selector3/1 -> Memory/1  "<Pilotiertes_Fahren_State>"
  Feedback_ADAS/1 -> Bus Selector3/1, Bus Selector4/1
  Memory/1 -> Logical Operator/1
  Logical Operator/1 -> ACC_User_Control/7(Enabled_Systems)
  Bus Selector3/2 -> Memory1/1  "<Emergency_Brake_State>"
  Memory1/1 -> Logical Operator/2
  Memory2/1 -> Logical Operator/3
  Bus Selector3/3 -> Memory2/1  "<Emergency_Steering_State>"

== system PC_Simulator_Lib/ADAS/Unser_Interface_ADAS/Emergency_Brake ==
  Feedback_ADAS : Inport
  Feedback_Simulationsumgebung : Inport  Port=2
  Bus Selector : BusSelector  OutputSignals=Driver_Interface.Emergency_Brake_Button
  Bus Selector1 : BusSelector  OutputSignals=Unser_Interface_ADAS.ACC.ACC_State,Unser_Interface_ADAS.Pilotiertes_Fahren.Pilotiertes_Fahren_State,Unser_Interface_ADAS.Emergency_Steering.Emergency_Steering_State
  Emergency_brake_HMI_model : Stateflow chart  TreatAsAtomicUnit=on
  Logical Operator : Logic  Operator=OR  Inputs=3  AllPortsSameDT=off  OutDataTypeStr=boolean
  Memory : Memory
  Memory1 : Memory
  Memory2 : Memory
  Mux1 : Mux  Inputs=2
  Pulse Generator : DiscretePulseGenerator  PulseType=Time based  Period=0.1  PulseWidth=50
  Emergency_Brake_State[bool] : Outport
  wires:
  Feedback_ADAS/1 -> Bus Selector1/1
  Emergency_brake_HMI_model/1(State) -> Emergency_Brake_State[bool]/1
  Bus Selector/1 -> Mux1/2  "<Emergency_Brake_Button>"
  Feedback_Simulationsumgebung/1 -> Bus Selector/1
  Pulse Generator/1 -> Mux1/1
  Mux1/1 -> Emergency_brake_HMI_model/Trigger
  Memory/1 -> Logical Operator/1
  Memory1/1 -> Logical Operator/2
  Logical Operator/1 -> Emergency_brake_HMI_model/1(Enabled_Systems)
  Bus Selector1/1 -> Memory/1  "<ACC_State>"
  Bus Selector1/2 -> Memory1/1  "<Pilotiertes_Fahren_State>"
  Memory2/1 -> Logical Operator/3
  Bus Selector1/3 -> Memory2/1  "<Emergency_Steering_State>"

== system PC_Simulator_Lib/ADAS/Unser_Interface_ADAS/Emergency_Steering ==
  Feedback_ADAS : Inport
  Feedback_Simulationsumgebung : Inport  Port=2
  Bus Selector : BusSelector  OutputSignals=Driver_Interface.Emergency_Steering_Button
  Bus Selector1 : BusSelector  OutputSignals=Unser_Interface_ADAS.ACC.ACC_State,Unser_Interface_ADAS.Pilotiertes_Fahren.Pilotiertes_Fahren_State,Unser_Interface_ADAS.Emergency_Brake
  Emergency_steer_HMI_model : Stateflow chart  TreatAsAtomicUnit=on
  Logical Operator : Logic  Operator=OR  Inputs=3  AllPortsSameDT=off  OutDataTypeStr=boolean
  Memory : Memory
  Memory1 : Memory
  Memory2 : Memory
  Mux1 : Mux  Inputs=2
  Pulse Generator : DiscretePulseGenerator  PulseType=Time based  Period=0.1  PulseWidth=50
  Emergency_Steering_State[bool] : Outport
  wires:
  Bus Selector1/2 -> Memory1/1  "<Pilotiertes_Fahren_State>"
  Bus Selector1/1 -> Memory/1  "<ACC_State>"
  Logical Operator/1 -> Emergency_steer_HMI_model/1(Enabled_Systems)
  Memory1/1 -> Logical Operator/2
  Memory/1 -> Logical Operator/1
  Mux1/1 -> Emergency_steer_HMI_model/Trigger
  Pulse Generator/1 -> Mux1/1
  Feedback_Simulationsumgebung/1 -> Bus Selector/1
  Bus Selector/1 -> Mux1/2  "<Emergency_Steering_Button>"
  Emergency_steer_HMI_model/1(State) -> Emergency_Steering_State[bool]/1
  Feedback_ADAS/1 -> Bus Selector1/1
  Memory2/1 -> Logical Operator/3
  Bus Selector1/3 -> Memory2/1  "<Emergency_Brake>"

== system PC_Simulator_Lib/ADAS/Unser_Interface_ADAS/Pilotiertes_Fahren ==
  Feedback_ADAS : Inport
  Feedback_Simulationsumgebung : Inport  Port=2
  Bus Selector : BusSelector  OutputSignals=Driver_Interface.Pilot_Button
  Bus Selector1 : BusSelector  OutputSignals=Unser_Interface_ADAS.ACC.ACC_State,Unser_Interface_ADAS.Emergency_Brake.Emergency_Brake_State,Unser_Interface_ADAS.Emergency_Steering.Emergency_Steering_State
  Bus Selector2 : BusSelector  OutputSignals=Driver_Interface.DNR,Driver_Interface.Acc_Pedal_norm,Driver_Interface.Brake_Pedal_norm
  Bus Selector4 : BusSelector  OutputSignals=Execution_ADAS.ADAS_controller_values.Acc_Pedal[norm],Execution_ADAS.ADAS_controller_values.Brake_Pedal[norm]
  Logical Operator : Logic  Operator=OR  Inputs=3  AllPortsSameDT=off  OutDataTypeStr=boolean
  Memory1 : Memory
  Memory2 : Memory
  Memory3 : Memory
  Mux1 : Mux  Inputs=2
  Pilotiertes_fahren_HMI_model : Stateflow chart  TreatAsAtomicUnit=on
  Pulse Generator : DiscretePulseGenerator  PulseType=Time based  Period=0.1  PulseWidth=50
  Pilotiertes_Fahren_State[bool] : Outport
  wires:
  Bus Selector4/1 -> Pilotiertes_fahren_HMI_model/5(Gas_Pedal_ACC)  "<Acc_Pedal[norm]>"
  Bus Selector4/2 -> Pilotiertes_fahren_HMI_model/6(Brake_Pedal_ACC)  "<Brake_Pedal[norm]>"
  Mux1/1 -> Pilotiertes_fahren_HMI_model/Trigger
  Pulse Generator/1 -> Mux1/1
  Bus Selector/1 -> Mux1/2  "<Pilot_Button>"
  Pilotiertes_fahren_HMI_model/1(State) -> Pilotiertes_Fahren_State[bool]/1
  Feedback_ADAS/1 -> Bus Selector1/1, Bus Selector4/1
  Bus Selector1/1 -> Memory1/1  "<ACC_State>"
  Memory1/1 -> Logical Operator/1
  Memory2/1 -> Logical Operator/2
  Logical Operator/1 -> Pilotiertes_fahren_HMI_model/1(Enabled_Systems)
  Bus Selector1/2 -> Memory2/1  "<Emergency_Brake_State>"
  Memory3/1 -> Logical Operator/3
  Bus Selector1/3 -> Memory3/1  "<Emergency_Steering_State>"
  Feedback_Simulationsumgebung/1 -> Bus Selector2/1, Bus Selector/1
  Bus Selector2/2 -> Pilotiertes_fahren_HMI_model/3(Gas_Pedal_User)  "<Acc_Pedal_norm>"
  Bus Selector2/1 -> Pilotiertes_fahren_HMI_model/2(Gearbox_State)  "<DNR>"
  Bus Selector2/3 -> Pilotiertes_fahren_HMI_model/4(Brake_Pedal_User)  "<Brake_Pedal_norm>"

== system PC_Simulator_Lib/Comunication_with_visualisation_Realtime/Maping_Block/Subsystem ==
  Vehicle_1_Vector : Inport
  Vehicle_2_Vector : Inport  Port=2
  Vehicle_3_Vector : Inport  Port=3
  Vehicle_4_Vector : Inport  Port=4
  Vehicle_5_Vector : Inport  Port=5
  Vehicle_6_Vector : Inport  Port=6
  Vehicle_7_Vector : Inport  Port=7
  Vehicle_8_Vector : Inport  Port=8
  Vehicle_9_Vector : Inport  Port=9
  Vehicle_10_Vector : Inport  Port=10
  Vehicle_11_Vector : Inport  Port=11
  Vehicle_12_Vector : Inport  Port=12
  Vehicle_13_Vector : Inport  Port=13
  Vehicle_14_Vector : Inport  Port=14
  Bus Creator : BusCreator  Inputs=14
  Bus Selector : BusSelector  OutputSignals=Vehicle_1_Vector.Vehicle_1_x[m],Vehicle_2_Vector.Vehicle_2_x[m],Vehicle_3_Vector.Vehicle_3_x[m],Vehicle_4_Vector3.Vehicle_4_x[m],Vehicle_5_Vector.Vehicle_5_x[m],Vehicle_6_Vector.Vehicle_6_x[m],Vehicle_7_Vector.Vehicle_7_x[m],Vehicle_8_Vector.Vehicle_8_x[m],Vehicle_9_Vector.Vehicle_9_x[m],Vehicle_10_Vector.Vehicle_10_x[m],Vehicle_11_Vector.Vehicle_11_x[m],Vehicle_12_Vector.Vehicle_12_x[m],Vehicle_13_Vector.Vehicle_13_x[m],Vehicle_14_Vector.Vehicle_14_x[m]
  Bus Selector1 : BusSelector  OutputSignals=Vehicle_1_Vector.Vehicle_1_y[m],Vehicle_2_Vector.Vehicle_2_y[m],Vehicle_3_Vector.Vehicle_3_y[m],Vehicle_4_Vector3.Vehicle_4_y[m],Vehicle_5_Vector.Vehicle_5_y[m],Vehicle_6_Vector.Vehicle_6_y[m],Vehicle_7_Vector.Vehicle_7_y[m],Vehicle_8_Vector.Vehicle_8_y[m],Vehicle_9_Vector.Vehicle_9_y[m],Vehicle_10_Vector.Vehicle_10_y[m],Vehicle_11_Vector.Vehicle_11_y[m],Vehicle_12_Vector.Vehicle_12_y[m],Vehicle_13_Vector.Vehicle_13_y[m],Vehicle_14_Vector.Vehicle_14_y[m]
  Bus Selector2 : BusSelector  OutputSignals=Vehicle_1_Vector.Vehicle_1_z[m],Vehicle_2_Vector.Vehicle_2_z[m],Vehicle_3_Vector.Vehicle_3_z[m],Vehicle_4_Vector3.Vehicle_4_z[m],Vehicle_5_Vector.Vehicle_5_z[m],Vehicle_6_Vector.Vehicle_6_z[m],Vehicle_7_Vector.Vehicle_7_z[m],Vehicle_8_Vector.Vehicle_8_z[m],Vehicle_9_Vector.Vehicle_9_z[m],Vehicle_10_Vector.Vehicle_10_z[m],Vehicle_11_Vector.Vehicle_11_z[m],Vehicle_12_Vector.Vehicle_12_z[m],Vehicle_13_Vector.Vehicle_13_z[m],Vehicle_14_Vector.Vehicle_14_z[m]
  Bus Selector3 : BusSelector  OutputSignals=Vehicle_1_Vector.Vehicle_1_Gear_Angle[deg],Vehicle_2_Vector.Vehicle_2_Gear_Angle[deg],Vehicle_3_Vector.Vehicle_3_Gear_Angle[deg],Vehicle_4_Vector3.Vehicle_4_Gear_Angle[deg],Vehicle_5_Vector.Vehicle_5_Gear_Angle[deg],Vehicle_6_Vector.Vehicle_6_Gear_Angle[deg],Vehicle_7_Vector.Vehicle_7_Gear_Angle[deg],Vehicle_8_Vector.Vehicle_8_Gear_Angle[deg],Vehicle_9_Vector.Vehicle_9_Gear_Angle[deg],Vehicle_10_Vector.Vehicle_10_Gear_Angle[deg],Vehicle_11_Vector.Vehicle_11_Gear_Angle[deg],Vehicle_12_Vector.Vehicle_12_Gear_Angle[deg],Vehicle_13_Vector.Vehicle_13_Gear_Angle[deg],Vehicle_14_Vector.Vehicle_14_Gear_Angle[deg]
  Bus Selector4 : BusSelector  OutputSignals=Vehicle_1_Vector.Vehicle_1_Wheels_Rotation_Angle[deg],Vehicle_2_Vector.Vehicle_2_Wheels_Rotation_Angle[deg],Vehicle_3_Vector.Vehicle_3_Wheels_Rotation_Angle[deg],Vehicle_4_Vector3.Vehicle_4_Wheels_Rotation_Angle[deg],Vehicle_5_Vector.Vehicle_5_Wheels_Rotation_Angle[deg],Vehicle_6_Vector.Vehicle_6_Wheels_Rotation_Angle[deg],Vehicle_7_Vector.Vehicle_7_Wheels_Rotation_Angle[deg],Vehicle_8_Vector.Vehicle_8_Wheels_Rotation_Angle[deg],Vehicle_9_Vector.Vehicle_9_Wheels_Rotation_Angle[deg],Vehicle_10_Vector.Vehicle_10_Wheels_Rotation_Angle[deg],Vehicle_11_Vector.Vehicle_11_Wheels_Rotation_Angle[deg],Vehicle_12_Vector.Vehicle_12_Wheels_Rotation_Angle[deg],Vehicle_13_Vector.Vehicle_13_Wheels_Rotation_Angle[deg],Vehicle_14_Vector.Vehicle_14_Wheels_Rotation_Angle[deg]
  Mux{,1..4} (5 alike) : Mux  Inputs=14
  Fellow_Vehicles_x_Vector_14[m] : Outport
  Fellow_Vehicles_y_Vector_14[m] : Outport  Port=2
  Fellow_Vehicles_z_Vector_14[m] : Outport  Port=3
  Fellow_Vehicles_Gear_Angle_Vector_14[deg] : Outport  Port=4
  Fellow_Vehicles_Wheel_Angle_Vector_14[deg] : Outport  Port=5
  wires:
  Vehicle_1_Vector/1 -> Bus Creator/1
  Vehicle_2_Vector/1 -> Bus Creator/2
  Vehicle_3_Vector/1 -> Bus Creator/3
  Vehicle_4_Vector/1 -> Bus Creator/4
  Vehicle_5_Vector/1 -> Bus Creator/5
  Vehicle_6_Vector/1 -> Bus Creator/6
  Vehicle_7_Vector/1 -> Bus Creator/7
  Vehicle_8_Vector/1 -> Bus Creator/8
  Vehicle_13_Vector/1 -> Bus Creator/13
  Vehicle_10_Vector/1 -> Bus Creator/10
  Vehicle_9_Vector/1 -> Bus Creator/9
  Vehicle_11_Vector/1 -> Bus Creator/11
  Vehicle_12_Vector/1 -> Bus Creator/12
  Vehicle_14_Vector/1 -> Bus Creator/14
  Bus Selector/8 -> Mux/8  "<Vehicle_8_x[m]>"
  Bus Selector/9 -> Mux/9  "<Vehicle_9_x[m]>"
  Bus Selector/7 -> Mux/7  "<Vehicle_7_x[m]>"
  Bus Selector/10 -> Mux/10  "<Vehicle_10_x[m]>"
  Bus Selector/6 -> Mux/6  "<Vehicle_6_x[m]>"
  Bus Selector/11 -> Mux/11  "<Vehicle_11_x[m]>"
  Bus Selector/5 -> Mux/5  "<Vehicle_5_x[m]>"
  Bus Selector/12 -> Mux/12  "<Vehicle_12_x[m]>"
  Bus Selector/4 -> Mux/4  "<Vehicle_4_x[m]>"
  Bus Selector/13 -> Mux/13  "<Vehicle_13_x[m]>"
  Bus Selector/3 -> Mux/3  "<Vehicle_3_x[m]>"
  Bus Selector/14 -> Mux/14  "<Vehicle_14_x[m]>"
  Bus Selector/2 -> Mux/2  "<Vehicle_2_x[m]>"
  Bus Selector/1 -> Mux/1  "<Vehicle_1_x[m]>"
  Bus Selector1/8 -> Mux1/8  "<Vehicle_8_y[m]>"
  Bus Selector1/9 -> Mux1/9  "<Vehicle_9_y[m]>"
  Bus Selector1/7 -> Mux1/7  "<Vehicle_7_y[m]>"
  Bus Selector1/10 -> Mux1/10  "<Vehicle_10_y[m]>"
  Bus Selector1/6 -> Mux1/6  "<Vehicle_6_y[m]>"
  Bus Selector1/11 -> Mux1/11  "<Vehicle_11_y[m]>"
  Bus Selector1/5 -> Mux1/5  "<Vehicle_5_y[m]>"
  Bus Selector1/12 -> Mux1/12  "<Vehicle_12_y[m]>"
  Bus Selector1/4 -> Mux1/4  "<Vehicle_4_y[m]>"
  Bus Selector1/13 -> Mux1/13  "<Vehicle_13_y[m]>"
  Bus Selector1/3 -> Mux1/3  "<Vehicle_3_y[m]>"
  Bus Selector1/14 -> Mux1/14  "<Vehicle_14_y[m]>"
  Bus Selector1/2 -> Mux1/2  "<Vehicle_2_y[m]>"
  Bus Selector1/1 -> Mux1/1  "<Vehicle_1_y[m]>"
  Bus Selector2/8 -> Mux2/8  "<Vehicle_8_z[m]>"
  Bus Selector2/9 -> Mux2/9  "<Vehicle_9_z[m]>"
  Bus Selector2/7 -> Mux2/7  "<Vehicle_7_z[m]>"
  Bus Selector2/10 -> Mux2/10  "<Vehicle_10_z[m]>"
  Bus Selector2/6 -> Mux2/6  "<Vehicle_6_z[m]>"
  Bus Selector2/11 -> Mux2/11  "<Vehicle_11_z[m]>"
  Bus Selector2/5 -> Mux2/5  "<Vehicle_5_z[m]>"
  Bus Selector2/12 -> Mux2/12  "<Vehicle_12_z[m]>"
  Bus Selector2/4 -> Mux2/4  "<Vehicle_4_z[m]>"
  Bus Selector2/13 -> Mux2/13  "<Vehicle_13_z[m]>"
  Bus Selector2/3 -> Mux2/3  "<Vehicle_3_z[m]>"
  Bus Selector2/14 -> Mux2/14  "<Vehicle_14_z[m]>"
  Bus Selector2/2 -> Mux2/2  "<Vehicle_2_z[m]>"
  Bus Selector2/1 -> Mux2/1  "<Vehicle_1_z[m]>"
  Bus Selector3/8 -> Mux3/8  "<Vehicle_8_Gear_Angle[deg]>"
  Bus Selector3/9 -> Mux3/9  "<Vehicle_9_Gear_Angle[deg]>"
  Bus Selector3/7 -> Mux3/7  "<Vehicle_7_Gear_Angle[deg]>"
  Bus Selector3/10 -> Mux3/10  "<Vehicle_10_Gear_Angle[deg]>"
  Bus Selector3/6 -> Mux3/6  "<Vehicle_6_Gear_Angle[deg]>"
  Bus Selector3/11 -> Mux3/11  "<Vehicle_11_Gear_Angle[deg]>"
  Bus Selector3/5 -> Mux3/5  "<Vehicle_5_Gear_Angle[deg]>"
  Bus Selector3/12 -> Mux3/12  "<Vehicle_12_Gear_Angle[deg]>"
  Bus Selector3/4 -> Mux3/4  "<Vehicle_4_Gear_Angle[deg]>"
  Bus Selector3/13 -> Mux3/13  "<Vehicle_13_Gear_Angle[deg]>"
  Bus Selector3/3 -> Mux3/3  "<Vehicle_3_Gear_Angle[deg]>"
  Bus Selector3/14 -> Mux3/14  "<Vehicle_14_Gear_Angle[deg]>"
  Bus Selector3/2 -> Mux3/2  "<Vehicle_2_Gear_Angle[deg]>"
  Bus Selector3/1 -> Mux3/1  "<Vehicle_1_Gear_Angle[deg]>"
  Bus Creator/1 -> Bus Selector4/1, Bus Selector3/1, Bus Selector2/1, Bus Selector1/1, Bus Selector/1
  Bus Selector4/8 -> Mux4/8  "<Vehicle_8_Wheels_Rotation_Angle[deg]>"
  Bus Selector4/9 -> Mux4/9  "<Vehicle_9_Wheels_Rotation_Angle[deg]>"
  Bus Selector4/7 -> Mux4/7  "<Vehicle_7_Wheels_Rotation_Angle[deg]>"
  Bus Selector4/10 -> Mux4/10  "<Vehicle_10_Wheels_Rotation_Angle[deg]>"
  Bus Selector4/6 -> Mux4/6  "<Vehicle_6_Wheels_Rotation_Angle[deg]>"
  Bus Selector4/11 -> Mux4/11  "<Vehicle_11_Wheels_Rotation_Angle[deg]>"
  Bus Selector4/5 -> Mux4/5  "<Vehicle_5_Wheels_Rotation_Angle[deg]>"
  Bus Selector4/12 -> Mux4/12  "<Vehicle_12_Wheels_Rotation_Angle[deg]>"
  Bus Selector4/4 -> Mux4/4  "<Vehicle_4_Wheels_Rotation_Angle[deg]>"
  Bus Selector4/13 -> Mux4/13  "<Vehicle_13_Wheels_Rotation_Angle[deg]>"
  Bus Selector4/3 -> Mux4/3  "<Vehicle_3_Wheels_Rotation_Angle[deg]>"
  Bus Selector4/14 -> Mux4/14  "<Vehicle_14_Wheels_Rotation_Angle[deg]>"
  Bus Selector4/2 -> Mux4/2  "<Vehicle_2_Wheels_Rotation_Angle[deg]>"
  Bus Selector4/1 -> Mux4/1  "<Vehicle_1_Wheels_Rotation_Angle[deg]>"
  Mux/1 -> Fellow_Vehicles_x_Vector_14[m]/1
  Mux1/1 -> Fellow_Vehicles_y_Vector_14[m]/1
  Mux2/1 -> Fellow_Vehicles_z_Vector_14[m]/1
  Mux3/1 -> Fellow_Vehicles_Gear_Angle_Vector_14[deg]/1
  Mux4/1 -> Fellow_Vehicles_Wheel_Angle_Vector_14[deg]/1

== system PC_Simulator_Lib/Comunication_with_visualisation_Realtime/Subsystem2/Subsystem ==
  In1 : Inport
  Constant9 : Constant  Value=Z_init
  Sum : Sum  Inputs=|++
  Out1 : Outport
  wires:
  In1/1 -> Sum/1
  Constant9/1 -> Sum/2
  Sum/1 -> Out1/1

== system PC_Simulator_Lib/Comunication_with_visualisation_Realtime/Subsystem2/Subsystem1 ==
  In1 : Inport
  Constant9 : Constant  Value=Z_init
  Sum : Sum  Inputs=|++
  Out1 : Outport
  wires:
  Sum/1 -> Out1/1
  Constant9/1 -> Sum/2
  In1/1 -> Sum/1

== system PC_Simulator_Lib/Comunication_with_visualisation_Realtime/Subsystem2/Subsystem10 ==
  In1 : Inport
  Constant9 : Constant  Value=Z_init
  Sum : Sum  Inputs=|++
  Out1 : Outport
  wires:
  Sum/1 -> Out1/1
  Constant9/1 -> Sum/2
  In1/1 -> Sum/1

== system PC_Simulator_Lib/Comunication_with_visualisation_Realtime/Subsystem2/Subsystem11 ==
  v[m|s] : Inport
  Gain : Gain  Gain=1/radiusWheel
  Integrator : Integrator
  Wheels_Rotation_Angle[rad] : Outport
  wires:
  Integrator/1 -> Wheels_Rotation_Angle[rad]/1
  v[m|s]/1 -> Gain/1
  Gain/1 -> Integrator/1

== system PC_Simulator_Lib/Comunication_with_visualisation_Realtime/Subsystem2/Subsystem12 ==
  v[m|s] : Inport
  Gain : Gain  Gain=1/radiusWheel
  Integrator : Integrator
  Wheels_Rotation_Angle[rad] : Outport
  wires:
  Gain/1 -> Integrator/1
  v[m|s]/1 -> Gain/1
  Integrator/1 -> Wheels_Rotation_Angle[rad]/1

== system PC_Simulator_Lib/Comunication_with_visualisation_Realtime/Subsystem2/Subsystem13 ==
  v[m|s] : Inport
  Gain : Gain  Gain=1/radiusWheel
  Integrator : Integrator
  Wheels_Rotation_Angle[rad] : Outport
  wires:
  Integrator/1 -> Wheels_Rotation_Angle[rad]/1
  v[m|s]/1 -> Gain/1
  Gain/1 -> Integrator/1

== system PC_Simulator_Lib/Comunication_with_visualisation_Realtime/Subsystem2/Subsystem14 ==
  v[m|s] : Inport
  Gain : Gain  Gain=1/radiusWheel
  Integrator : Integrator
  Wheels_Rotation_Angle[rad] : Outport
  wires:
  Gain/1 -> Integrator/1
  v[m|s]/1 -> Gain/1
  Integrator/1 -> Wheels_Rotation_Angle[rad]/1

== system PC_Simulator_Lib/Comunication_with_visualisation_Realtime/Subsystem2/Subsystem15 ==
  v[m|s] : Inport
  Gain : Gain  Gain=1/radiusWheel
  Integrator : Integrator
  Wheels_Rotation_Angle[rad] : Outport
  wires:
  Integrator/1 -> Wheels_Rotation_Angle[rad]/1
  v[m|s]/1 -> Gain/1
  Gain/1 -> Integrator/1

== system PC_Simulator_Lib/Comunication_with_visualisation_Realtime/Subsystem2/Subsystem16 ==
  v[m|s] : Inport
  Gain : Gain  Gain=1/radiusWheel
  Integrator : Integrator
  Wheels_Rotation_Angle[rad] : Outport
  wires:
  Gain/1 -> Integrator/1
  v[m|s]/1 -> Gain/1
  Integrator/1 -> Wheels_Rotation_Angle[rad]/1
